simulink model "P2"  (R2020b)
settings: Solver=VariableStepAuto  StartTime=0.0  StopTime=10.0  RelTol=1e-3
settings Model: Creator=albac  LastModifiedBy=albac

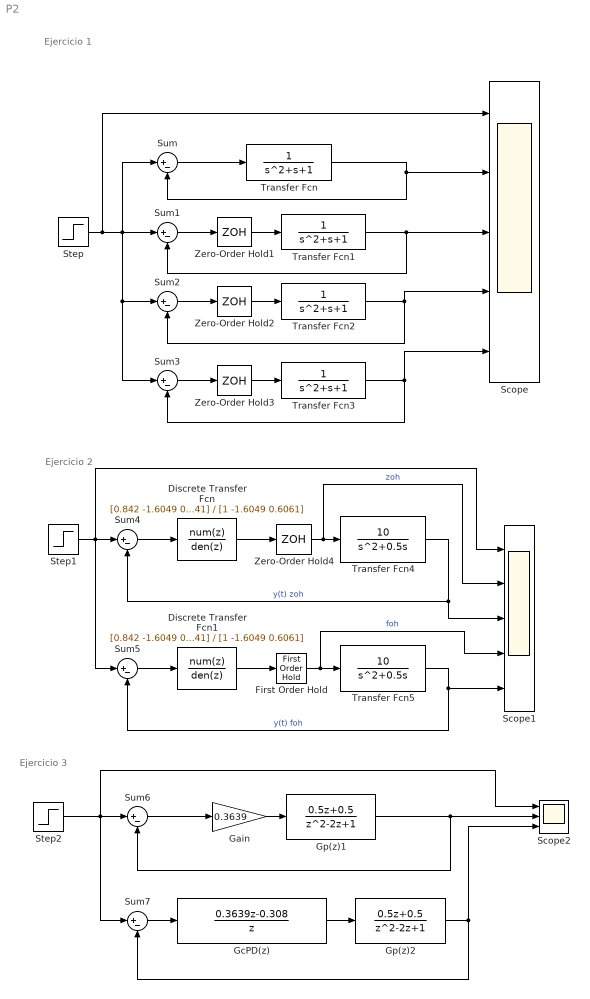
== system P2 ==
  note: Ejercicio 3
  note: Ejercicio 1
  note: Ejercicio 2
  Discrete Transfer Fcn : DiscreteTransferFcn  Numerator=[0.842 -1.6049 0.7641]  Denominator=[1 -1.6049 0.6061]  SampleTime=0.1
  Discrete Transfer Fcn1 : DiscreteTransferFcn  Numerator=[0.842 -1.6049 0.7641]  Denominator=[1 -1.6049 0.6061]  SampleTime=0.1
  First Order Hold : FirstOrderHold  ErrorTolerance=inf
  Gain : Gain  Gain=0.3639
  GcPD(z) : DiscreteTransferFcn  Numerator=[0.3639 -0.308]  Denominator=[1 0]
  Gp(z)1 : DiscreteTransferFcn  Numerator=[0.5 0.5]  Denominator=[1 -2 1]  SampleTime=0.1
  Gp(z)2 : DiscreteTransferFcn  Numerator=[0.5 0.5]  Denominator=[1 -2 1]  SampleTime=0.1
  Scope : Scope  NumInputPorts=5
  Scope1 : Scope  NumInputPorts=5
  Scope2 : Scope  NumInputPorts=3
  Step : Step  Time=0  SampleTime=0
  Step1 : Step  Time=0  SampleTime=0
  Step2 : Step  Time=0  SampleTime=0
  Sum{,1..7} (8 alike) : Sum  Inputs=|+-
  Transfer Fcn{,1..3} (4 alike) : TransferFcn  Denominator=[1 1 1]
  Transfer Fcn4 : TransferFcn  Numerator=[10]  Denominator=[1 0.5 0]
  Transfer Fcn5 : TransferFcn  Numerator=[10]  Denominator=[1 0.5 0]
  Zero-Order Hold1 : ZeroOrderHold  SampleTime=0.01
  Zero-Order Hold2 : ZeroOrderHold  SampleTime=0.1
  Zero-Order Hold3 : ZeroOrderHold
  Zero-Order Hold4 : ZeroOrderHold  SampleTime=0.1
  wires:
  Sum/1 -> Transfer Fcn/1
  Transfer Fcn/1 -> Sum/2, Scope/2
  Step/1 -> Scope/1, Sum3/1, Sum2/1, Sum1/1, Sum/1
  Zero-Order Hold1/1 -> Transfer Fcn1/1
  Transfer Fcn1/1 -> Sum1/2, Scope/3
  Sum1/1 -> Zero-Order Hold1/1
  Sum2/1 -> Zero-Order Hold2/1
  Zero-Order Hold2/1 -> Transfer Fcn2/1
  Transfer Fcn2/1 -> Sum2/2, Scope/4
  Transfer Fcn3/1 -> Scope/5, Sum3/2
  Zero-Order Hold3/1 -> Transfer Fcn3/1
  Sum3/1 -> Zero-Order Hold3/1
  Step1/1 -> Sum5/1, Scope1/1, Sum4/1
  Zero-Order Hold4/1 -> Scope1/2, Transfer Fcn4/1  "zoh"
  Transfer Fcn4/1 -> Sum4/2, Scope1/3  "y(t) zoh"
  Sum4/1 -> Discrete Transfer Fcn/1
  Discrete Transfer Fcn/1 -> Zero-Order Hold4/1
  Sum5/1 -> Discrete Transfer Fcn1/1
  Discrete Transfer Fcn1/1 -> First Order Hold/1
  First Order Hold/1 -> Scope1/4, Transfer Fcn5/1  "foh"
  Transfer Fcn5/1 -> Scope1/5, Sum5/2  "y(t) foh"
  Gain/1 -> Gp(z)1/1
  Sum6/1 -> Gain/1
  Gp(z)1/1 -> Scope2/2, Sum6/2
  Sum7/1 -> GcPD(z)/1
  Step2/1 -> Scope2/1, Sum7/1, Sum6/1
  GcPD(z)/1 -> Gp(z)2/1
  Gp(z)2/1 -> Sum7/2, Scope2/3
